simulink model "Prova_es3_sim"  (R2022b)
settings: Solver=VariableStepAuto  StartTime=0.0  StopTime=10.0  RelTol=1e-3
values from neighbouring files (symbols this model uses):
  A0 = sysC_d.A(2,2)-(L*sysC_d.A(1,2))    [Prova_es2.m]    (also in Prova_es2_MIK.m = sysC_d.A-(L*sysC_d.C))
  B0 = [sysC_d.B(2)-(L*sysC_d.B(1)) (A0*L)-sysC_d.A(2,1)-(L*sysC_d.A(1,1))]    [Prova_es2.m]    (also in Prova_es2_MIK.m = [sysC_d.B L])
  C0 = [0;1]    [Prova_es2.m]    (also in Prova_es2_MIK.m = eye(2))
  D0 = [0 1; 0 L]    [Prova_es2.m]    (also in Prova_es2_MIK.m = zeros(2))
  Nu = X(3)    [Prova_es2.m]    (also in Prova_es2_MIK.m)
  Nx = X(1:2)    [Prova_es2.m]    (also in Prova_es2_MIK.m)
undefined symbols (not defined in the file or in its folder): den, DiscIntNeverNeededParam, intg, num, Ts
settings Model: Creator=marcoverri  LastModifiedBy=emanuelevitetta

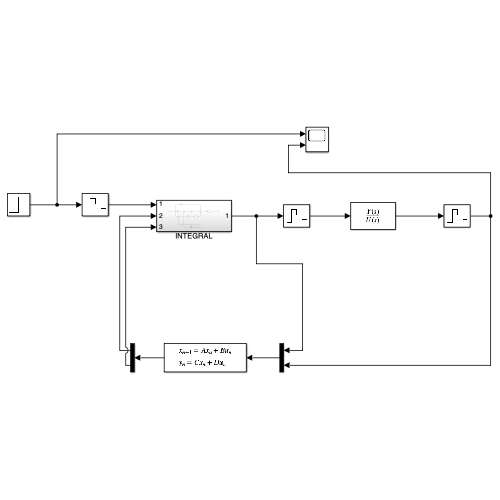
[thumbnail: Simulink's stored preview of the top-level diagram]
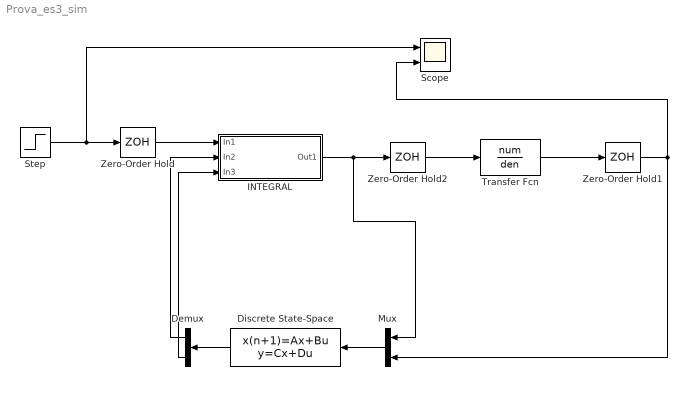
== system Prova_es3_sim ==
  Demux : Demux  Outputs=2
  Discrete State-Space : DiscreteStateSpace  A=A0  B=B0  C=C0  D=D0  SampleTime=Ts
  INTEGRAL : Subsystem
  Mux : Mux  Inputs=2
  Scope : Scope  NumInputPorts=2
  Step : Step  SampleTime=0
  Transfer Fcn : TransferFcn  Numerator=num  Denominator=den
  Zero-Order Hold : ZeroOrderHold  SampleTime=Ts
  Zero-Order Hold1 : ZeroOrderHold  SampleTime=Ts
  Zero-Order Hold2 : ZeroOrderHold  SampleTime=Ts
  wires:
  Step/1 -> Scope/1, Zero-Order Hold/1
  Zero-Order Hold/1 -> INTEGRAL/1(In1)
  INTEGRAL/1(Out1) -> Zero-Order Hold2/1, Mux/1
  Zero-Order Hold2/1 -> Transfer Fcn/1
  Transfer Fcn/1 -> Zero-Order Hold1/1
  Zero-Order Hold1/1 -> Mux/2, Scope/2
  Mux/1 -> Discrete State-Space/1
  Discrete State-Space/1 -> Demux/1
  Demux/1 -> INTEGRAL/2(In2)
  Demux/2 -> INTEGRAL/3(In3)

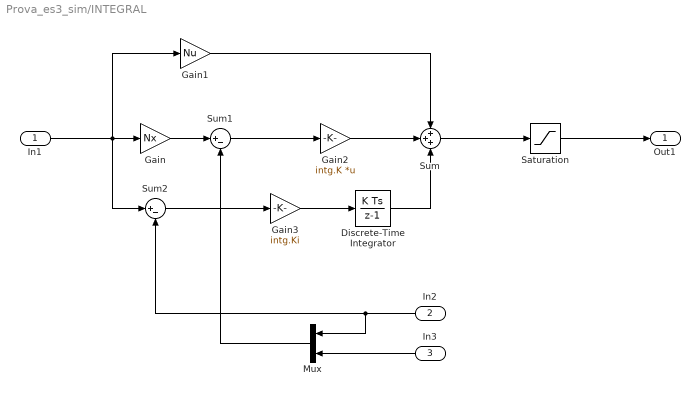
== system Prova_es3_sim/INTEGRAL ==
  In1 : Inport
  In2 : Inport  Port=2
  In3 : Inport  Port=3
  Discrete-Time Integrator : DiscreteIntegrator  SampleTime=Ts  ICPrevOutput=DiscIntNeverNeededParam  ICPrevScaledInput=DiscIntNeverNeededParam
  Gain : Gain  Gain=Nx
  Gain1 : Gain  Gain=Nu
  Gain2 : Gain  Gain=intg.K  Multiplication=Matrix(K*u)
  Gain3 : Gain  Gain=intg.Ki
  Mux : Mux  Inputs=2
  Saturation : Saturate  UpperLimit=10  LowerLimit=-10
  Sum : Sum  Inputs=+++
  Sum1 : Sum  Inputs=|+-
  Sum2 : Sum  Inputs=|+-
  Out1 : Outport
  wires:
  In1/1 -> Sum2/1, Gain1/1, Gain/1
  Saturation/1 -> Out1/1
  Sum/1 -> Saturation/1
  Gain2/1 -> Sum/2
  Gain1/1 -> Sum/1
  Gain3/1 -> Discrete-Time Integrator/1
  Discrete-Time Integrator/1 -> Sum/3
  Sum1/1 -> Gain2/1
  Gain/1 -> Sum1/1
  Sum2/1 -> Gain3/1
  In3/1 -> Mux/2
  In2/1 -> Sum2/2, Mux/1
  Mux/1 -> Sum1/2
